simulink model "digitalSMC_bicycle_sim"  (R2026a)
settings: Solver=FixedStepAuto  StopTime=10  FixedStep=Ts  MaxStep=0.01
values from neighbouring files (symbols this model uses):
  A_ = [eye(1),-Cd*Ad ... (first row only)    [digitalSMC_bicycle.m]
  Bd = Bd_and_Ed(:,1)    [digitalSMC_bicycle.m]
  Cd = C    [digitalSMC_bicycle.m]
  Ed = Bd_and_Ed(:,2)    [digitalSMC_bicycle.m]
  etta = 0.9    [digitalSMC_bicycle.m]
  I = eye(3)    [digitalSMC_bicycle.m]
  invSB_ = inv(SB_)    [digitalSMC_bicycle.m]
  S = dlqr(A_,B_,Q,R),    [digitalSMC_bicycle.m]
  ToRad = pi/180    (= 0.0174532925199)    [digitalSMC_bicycle.m]
  Ts = 0.005    [digitalSMC_bicycle.m]
undefined symbols (not defined in the file or in its folder): Ad
settings Model: Creator=Tomino Shun
settings SolverCC: ZeroCrossAlgorithm=Adaptive
settings DebuggingCC: IgnoredZcDiagnostic=none

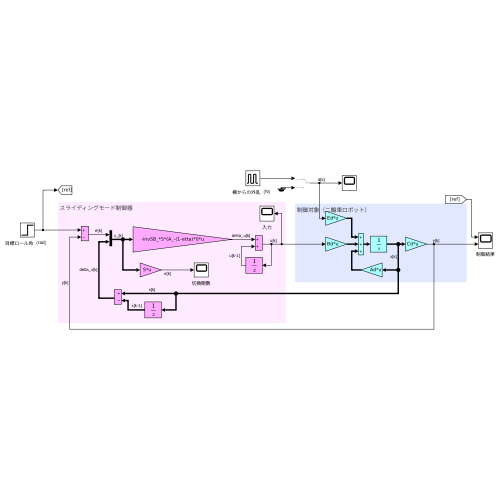
[thumbnail: Simulink's stored preview of the top-level diagram]
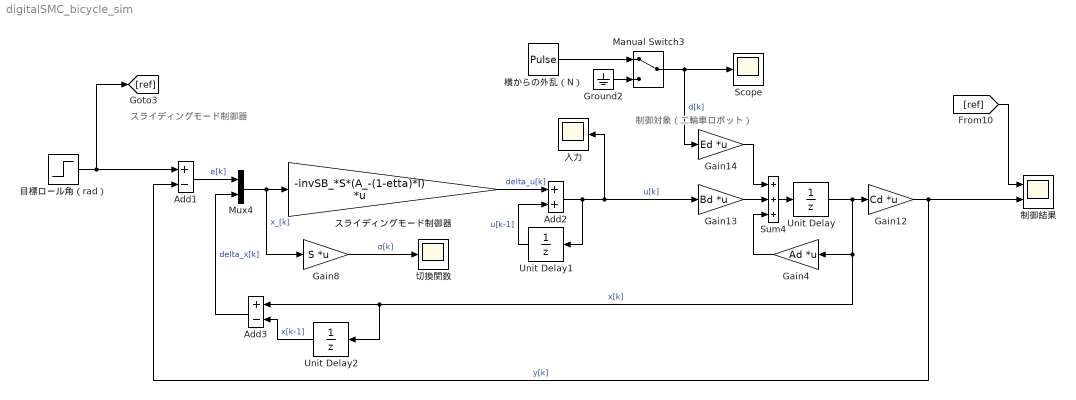
== system digitalSMC_bicycle_sim ==
  note: スライディングモード制御器
  note: 制御対象（二輪車ロボット）
  Add1 : Sum  Inputs=+-
  Add2 : Sum
  Add3 : Sum  Inputs=+-
  Gain12 : Gain  Gain=Cd  Multiplication=Matrix(K*u)
  Gain13 : Gain  Gain=Bd  Multiplication=Matrix(K*u)
  Gain14 : Gain  Gain=Ed  Multiplication=Matrix(K*u)
  Gain4 : Gain  Gain=Ad  Multiplication=Matrix(K*u)
  Gain8 : Gain  Gain=S  Multiplication=Matrix(K*u)
  Ground2 : Ground
  Manual Switch3 : ManualSwitch
  Mux4 : Mux  Inputs=2
  Scope : Scope
      settings: TimeUnits=Metric (based on Time Span)  ActiveDisplayYMinimum=-0.12499999999999997  ActiveDisplayYMaximum=1.125  YLabel=外乱(N)
  Sum4 : Sum  Inputs=+++
  Unit Delay : UnitDelay  InitialCondition=[0;0]  SampleTime=Ts
  Unit Delay1 : UnitDelay  SampleTime=Ts
  Unit Delay2 : UnitDelay  SampleTime=Ts
  スライディングモード制御器 : Gain  Gain=-invSB_*S*(A_-(1-etta)*I)  Multiplication=Matrix(K*u)
  入力 : Scope
      settings: ActiveDisplayYMinimum=-0.65239726564794909  ActiveDisplayYMaximum=0.54563132279381  DataLoggingVariableName=ScopeData3
  切換関数 : Scope
      settings: ActiveDisplayYMinimum=-0.0633847691253238  ActiveDisplayYMaximum=0.049457865467814194
  制御結果 : Scope  NumInputPorts=2
      settings: TimeUnits=Metric (based on Time Span)  ActiveDisplayYMinimum=-0.022040680810068193  ActiveDisplayYMaximum=0.19836612729061376  YLabel=ロール角(rad)  DataLoggingVariableName=ScopeData2
  横からの外乱（N） : DiscretePulseGenerator  PulseType=Time based  Period=10  PulseWidth=10  PhaseDelay=5
  目標ロール角（rad） : Step  Time=2  FinalValue=10*ToRad  SampleTime=Ts
  wires:
  Ground2/1 -> Manual Switch3/2
  横からの外乱（N）/1 -> Manual Switch3/1
  Gain4/1 -> Sum4/3
  Sum4/1 -> Unit Delay/1
  Unit Delay/1 -> Unit Delay2/1, Add3/1, Gain4/1, Gain12/1  "x[k]"
  Gain13/1 -> Sum4/2
  Gain14/1 -> Sum4/1
  Manual Switch3/1 -> Scope/1, Gain14/1  "d[k]"
  目標ロール角（rad）/1 -> [ref], Add1/1
  Mux4/1 -> Gain8/1, スライディングモード制御器/1  "x_[k]"
  Add1/1 -> Mux4/1  "e[k]"
  Gain8/1 -> 切換関数/1  "σ[k]"
  [ref] -> 制御結果/1
  Gain12/1 -> 制御結果/2, Add1/2  "y[k]"
  スライディングモード制御器/1 -> Add2/1  "delta_u[k]"
  Add2/1 -> Gain13/1, 入力/1, Unit Delay1/1  "u[k]"
  Unit Delay1/1 -> Add2/2  "u[k-1]"
  Add3/1 -> Mux4/2  "delta_x[k]"
  Unit Delay2/1 -> Add3/2  "x[k-1]"
